simulink library "ESTS_LSM_DYN"  (R2023b)
settings: Solver=VariableStepAuto  StartTime=0.0  StopTime=10.0  RelTol=1e-3
undefined symbols (not defined in the file): DiscIntNeverNeededParam, p_CrnrgStfnFr_Nprad, p_CrnrgStfnRe_Nprad, p_JzVeh_kgm2
libraries: VUT_lib x5
settings Model: Creator=blatak  LastModifiedBy=blatak

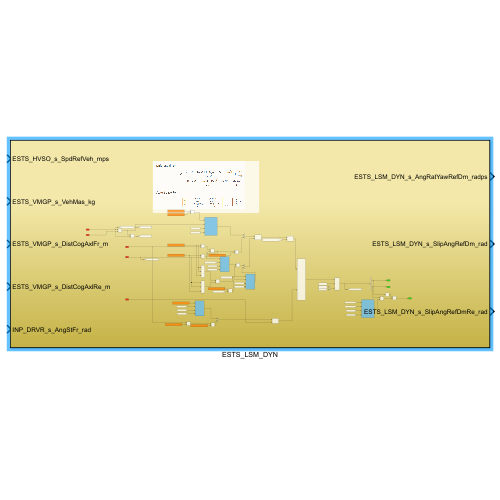
[thumbnail: Simulink's stored preview of the top-level diagram]
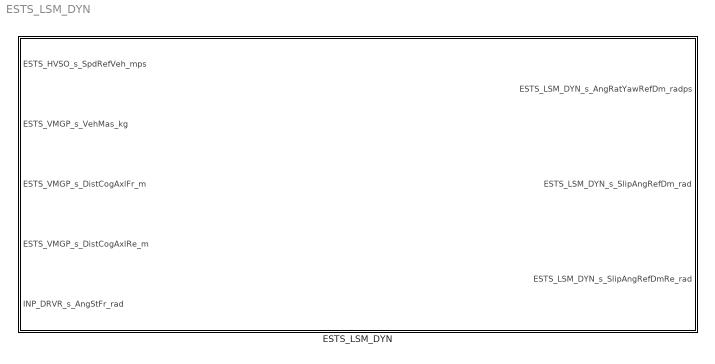
== system ESTS_LSM_DYN ==
  ESTS_LSM_DYN : Subsystem

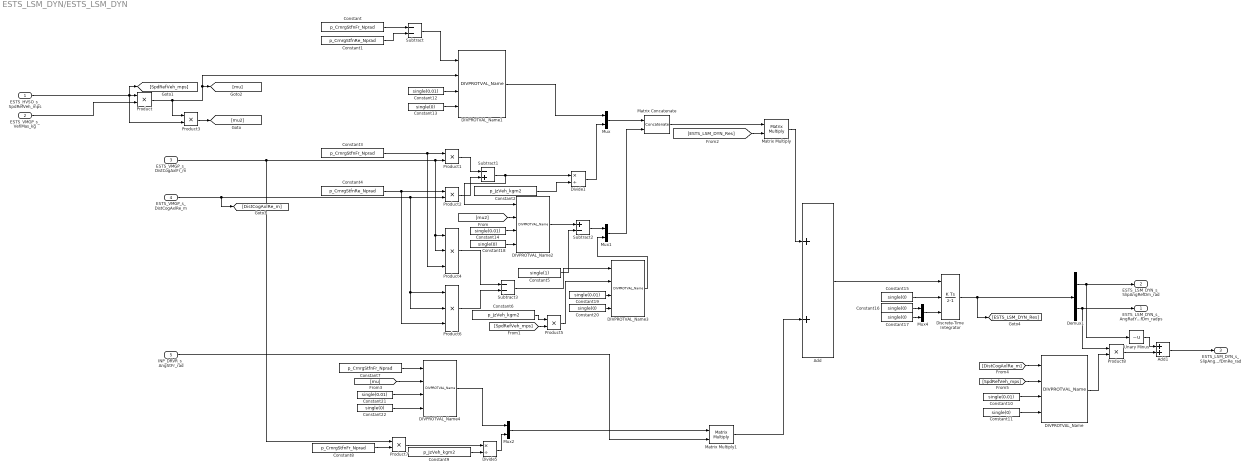
== system ESTS_LSM_DYN/ESTS_LSM_DYN ==
  ESTS_HVSO_s_SpdRefVeh_mps : Inport  Description=Estimated reference vehicle speed
  ESTS_VMGP_s_VehMas_kg : Inport  Description=Vehicle mass  Port=2
  ESTS_VMGP_s_DistCogAxlFr_m : Inport  Description=X distance from front axle (wheel center) to cog  Port=3
  ESTS_VMGP_s_DistCogAxlRe_m : Inport  Description=X distance from rear axle (wheel center) to cog  Port=4
  INP_DRVR_s_AngStFr_rad : Inport  Description=|  Port=5
      | Steering wheel angle front - calculated as an average FL and FR,
      | used for single track model, later more sophisticated calculation method needed 
      | than only an average
  Add : Sum
  Add1 : Sum
  Constant{,3,7..8} (4 alike) : Constant  Value=p_CrnrgStfnFr_Nprad
  Constant1 : Constant  Value=p_CrnrgStfnRe_Nprad
  Constant{10,12,14,19,21} (5 alike) : Constant  Value=single(0.01)
  Constant{11,13,15..18,20,22} (8 alike) : Constant  Value=single(0)
  Constant2 : Constant  Value=p_JzVeh_kgm2
  Constant4 : Constant  Value=p_CrnrgStfnRe_Nprad
  Constant5 : Constant  Value=single(1)
  Constant6 : Constant  Value=p_JzVeh_kgm2
  Constant9 : Constant  Description=Vehicle yaw moment of inertia  Value=p_JzVeh_kgm2
  DIVPROTVAL_Name{,1..4} (5 alike) : VUT_lib/DIVPROTVAL_Name  SystemSampleTime=-1  VariantActivationTime=update diagram  AllowFlexibleInterface=on  Latency=0  AutoFrameSizeCalculation=off
  Demux1 : Demux  Outputs=2
  Discrete-Time Integrator : DiscreteIntegrator  ExternalReset=rising  InitialConditionSource=external  SampleTime=-1  ICPrevOutput=DiscIntNeverNeededParam  ICPrevScaledInput=DiscIntNeverNeededParam
  Divide1 : Product  Inputs=*/  RndMeth=Zero  SaturateOnIntegerOverflow=on
  Divide5 : Product  Inputs=*/  RndMeth=Zero  SaturateOnIntegerOverflow=on
  Matrix Concatenate : Concatenate  Mode=Multidimensional array  ConcatenateDimension=2
  Matrix Multiply : Product  Multiplication=Matrix(*)
  Matrix Multiply1 : Product  Multiplication=Matrix(*)
  Mux{,1..2,4} (4 alike) : Mux  Inputs=2
  Product{,1..3,5,7..8} (7 alike) : Product
  Product4 : Product  Inputs=3
  Product6 : Product  Inputs=3
  Subtract : Sum  Inputs=--
  Subtract1 : Sum  Inputs=-+
  Subtract2 : Sum  Inputs=+-
  Subtract3 : Sum  Inputs=--
  Unary Minus : UnaryMinus
  ESTS_LSM_DYN_s_AngRatYawRefDm_radps : Outport  Description=Reference yaw velocity from dynamic single track model
  ESTS_LSM_DYN_s_SlipAngRefDm_rad : Outport  Description=Reference slip angle in cog from dynamic single track model  Port=2
  ESTS_LSM_DYN_s_SlipAngRefDmRe_rad : Outport  Description=Reference slip angle on rear axle from dynamic single track model  Port=3
  wires:
  [SpdRefVeh_mps] -> DIVPROTVAL_Name/2
  ESTS_VMGP_s_DistCogAxlRe_m/1 -> [DistCogAxlRe_m], Product6/2, Product6/1, Product2/2
  Mux/1 -> Matrix Concatenate/1
  ESTS_VMGP_s_DistCogAxlFr_m/1 -> Product7/1, Product4/2, Product4/1, Product1/2
  Matrix Multiply1/1 -> Add/2
  [DistCogAxlRe_m] -> DIVPROTVAL_Name/1
  Product/1 -> Product3/1, DIVPROTVAL_Name1/2, [mu]
  [mu2] -> DIVPROTVAL_Name2/2
  Product7/1 -> Divide5/1
  Add/1 -> Discrete-Time Integrator/1
  Unary Minus/1 -> Add1/1
  Constant19/1 -> DIVPROTVAL_Name3/3
  Subtract2/1 -> Mux1/1
  Subtract/1 -> DIVPROTVAL_Name1/1
  Demux1/2 -> ESTS_LSM_DYN_s_AngRatYawRefDm_radps/1, Product8/1
  Mux1/1 -> Matrix Concatenate/2
  ESTS_VMGP_s_VehMas_kg/1 -> Product/2
  Product4/1 -> Subtract3/1
  Constant11/1 -> DIVPROTVAL_Name/4
  Constant1/1 -> Subtract/2
  Constant10/1 -> DIVPROTVAL_Name/3
  Matrix Multiply/1 -> Add/1
  Add1/1 -> ESTS_LSM_DYN_s_SlipAngRefDmRe_rad/1
  Subtract3/1 -> DIVPROTVAL_Name3/1
  Demux1/1 -> ESTS_LSM_DYN_s_SlipAngRefDm_rad/1, Unary Minus/1
  INP_DRVR_s_AngStFr_rad/1 -> Matrix Multiply1/2
  Constant16/1 -> Mux4/1
  Constant13/1 -> DIVPROTVAL_Name1/4
  Product8/1 -> Add1/2
  Constant22/1 -> DIVPROTVAL_Name4/4
  Constant21/1 -> DIVPROTVAL_Name4/3
  Discrete-Time Integrator/1 -> Demux1/1, [ESTS_LSM_DYN_Res]
  [mu] -> DIVPROTVAL_Name4/2
  DIVPROTVAL_Name3/1 -> Mux1/2
  Subtract1/1 -> DIVPROTVAL_Name2/1, Divide1/1
  Constant3/1 -> Product4/3, Product1/1
  Constant18/1 -> DIVPROTVAL_Name2/4
  Matrix Concatenate/1 -> Matrix Multiply/1
  DIVPROTVAL_Name2/1 -> Subtract2/1
  DIVPROTVAL_Name/1 -> Product8/2
  [SpdRefVeh_mps] -> Product5/2
  Product5/1 -> DIVPROTVAL_Name3/2
  Constant12/1 -> DIVPROTVAL_Name1/3
  Constant14/1 -> DIVPROTVAL_Name2/3
  Constant4/1 -> Product6/3, Product2/1
  Mux2/1 -> Matrix Multiply1/1
  [ESTS_LSM_DYN_Res] -> Matrix Multiply/2
  Product1/1 -> Subtract1/1
  Constant/1 -> Subtract/1
  ESTS_HVSO_s_SpdRefVeh_mps/1 -> [SpdRefVeh_mps], Product3/2, Product/1
  Mux4/1 -> Discrete-Time Integrator/3
  Constant5/1 -> Subtract2/2
  Divide1/1 -> Mux/2
  Product2/1 -> Subtract1/2
  Constant7/1 -> DIVPROTVAL_Name4/1
  DIVPROTVAL_Name1/1 -> Mux/1
  Divide5/1 -> Mux2/2
  Constant17/1 -> Mux4/2
  Constant20/1 -> DIVPROTVAL_Name3/4
  Constant6/1 -> Product5/1
  Product6/1 -> Subtract3/2
  Constant15/1 -> Discrete-Time Integrator/2
  Constant2/1 -> Divide1/2
  DIVPROTVAL_Name4/1 -> Mux2/1
  Product3/1 -> [mu2]
  Constant8/1 -> Product7/2
  Constant9/1 -> Divide5/2
